simulink model "STH_LinearTF"  (R2020b)
settings: Solver=FixedStepAuto  StartTime=0.0  StopTime=1800  FixedStep=5  RelTol=1e-3
values from neighbouring files (symbols this model uses):
  Ts = 51.67    [Exp2_STH.m]
libraries: cstblocks x4
settings Model: Creator=franc  LastModifiedBy=franc

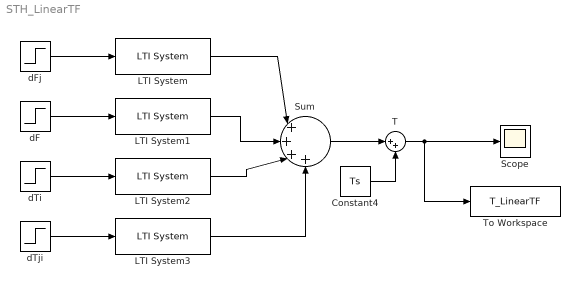
== system STH_LinearTF ==
  "            T" : Sum  Inputs=|++
  Constant4 : Constant  Value=Ts
  LTI System : cstblocks/LTI System  sys=G  IC=[]
  LTI System1 : cstblocks/LTI System  sys=Gd1  IC=[]
  LTI System2 : cstblocks/LTI System  sys=Gd2  IC=[]
  LTI System3 : cstblocks/LTI System  sys=Gd3  IC=[]
  Scope : Scope
  Sum : Sum  Inputs=|++++
  To Workspace : ToWorkspace  VariableName=T_LinearTF  SaveFormat=Timeseries  SampleTime=-1
  dF : Step  Time=0  After=0  SampleTime=0
  dFj : Step  Time=0  After=4.72e-5  SampleTime=0
  dTi : Step  Time=0  After=0  SampleTime=0
  dTji : Step  Time=0  After=0  SampleTime=0
  wires:
  dFj/1 -> LTI System/1
  dF/1 -> LTI System1/1
  dTi/1 -> LTI System2/1
  dTji/1 -> LTI System3/1
  LTI System1/1 -> Sum/2
  LTI System2/1 -> Sum/3
  LTI System/1 -> Sum/1
  LTI System3/1 -> Sum/4
  Sum/1 -> "            T"/1
  Constant4/1 -> "            T"/2
  "            T"/1 -> Scope/1, To Workspace/1
